simulink model "part2"  (R2018b)
settings: Solver=FixedStepDiscrete  StartTime=0.0  StopTime=150  RelTol=1e-3
settings Model: Creator=w_chenxu  LastModifiedBy=w_chenxu

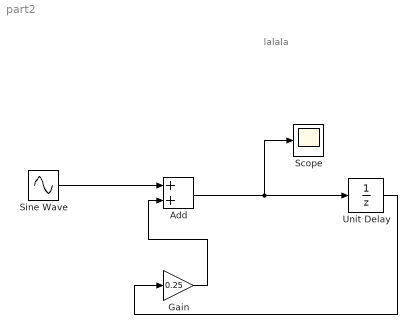
== system part2 ==
  note: lalala
  Add : Sum
  Gain : Gain  Gain=0.25
  Scope : Scope
  Sine Wave : Sin  Frequency=2*pi*(1/150)  SampleTime=5
  Unit Delay : UnitDelay  SampleTime=-1
  wires:
  Sine Wave/1 -> Add/1
  Gain/1 -> Add/2
  Add/1 -> Scope/1, Unit Delay/1
  Unit Delay/1 -> Gain/1
